simulink model "mrefrobotarm_modified_previous_y_previous_ref"  (R2018b)
settings: Solver=FixedStepAuto  StartTime=0.0  StopTime=60  RelTol=1e-3  AbsTol=1e-6
undefined symbols (not defined in the file or in its folder): sfunxy2
libraries: neural x301, simulink x1
(part 8 of 10)

== system mrefrobotarm_modified_previous_y_previous_ref/Feed-Forward Neural Network5/Layer 2/Delays 1 ==
  "p{2}" : Inport  PortDimensions=64
      mask Display: e = 0.06;c1 = [120 230 180]/255;c2 = ([120 230 180]+0)/(256+128);c3 = ([120 230 180]+128)/(256+128);patch([0 1 1 0],[0 0 1 1],c1);patch([0 1 1 1-e 1-e 0+e],[0 0 1 1-e 0+e 0+e],c2);patch([0 0 1 1-e 0+e 0+e],[0 1 1 1-e 1-e 0+e],c3);plot([0 1 1 0 0],[0 0 1 1 0]);
  mux : Mux  Inputs=1
      mask Display: e = 0.06;c1 = [120 150 230]/255;c2 = ([120 150 230]+0)/383;c3 = ([120 150 230]+128)/383;patch([0 1 1 0],[0 0 1 1],c1);patch([0 1 1 1-e 1-e 0+e],[0 0 1 1-e 0+e 0+e],c2);patch([0 0 1 1-e 0+e 0+e],[0 1 1 1-e 1-e 0+e],c3);plot([0 1 1 0 0],[0 0 1 1 0]);disp('Mux')
  "pd{2,1}" : Outport
      mask Display: e = 0.06;c1 = [120 230 180]/255;c2 = ([120 230 180]+0)/(256+128);c3 = ([120 230 180]+128)/(256+128);patch([0 1 1 0],[0 0 1 1],c1);patch([0 1 1 1-e 1-e 0+e],[0 0 1 1-e 0+e 0+e],c2);patch([0 0 1 1-e 0+e 0+e],[0 1 1 1-e 1-e 0+e],c3);plot([0 1 1 0 0],[0 0 1 1 0]);
  wires:
  "p{2}"/1 -> mux/1
  mux/1 -> "pd{2,1}"/1

== system mrefrobotarm_modified_previous_y_previous_ref/Feed-Forward Neural Network5/Layer 2/LW{2,1} ==
  "ad{2,1}" : Inport  PortDimensions=64
      mask Display: e = 0.06;c1 = [120 230 180]/255;c2 = ([120 230 180]+0)/(256+128);c3 = ([120 230 180]+128)/(256+128);patch([0 1 1 0],[0 0 1 1],c1);patch([0 1 1 1-e 1-e 0+e],[0 0 1 1-e 0+e 0+e],c2);patch([0 0 1 1-e 0+e 0+e],[0 1 1 1-e 1-e 0+e],c3);plot([0 1 1 0 0],[0 0 1 1 0]);
  "IW{2,1}(1,:)'" : Constant  Value=[0.1342055289137980278457717986384523101150989532470703125;-0.286006926010919482195049567962996661663055419921875;-0.189584300225614732493539804636384360492229461669921875;-0.09398592052439856681100849300491972826421260833740234375;-0.0188392157778938286460945761291441158391535282135009765625;-0.1923501339435728929583291346716578118503093719482421875;0.238509813288973526734793040304793976247310638427734375;0.11951515110633703642406544531695544719696044921875;0.204186071860302853497870501087163574993610382080078125;0.5849411103638357811718151424429379403591156005859375;0.1950905033324568937924681222284561954438686370849609375;0.1062361826918395701913055972909205593168735504150390625;-0.200821513449202626588885323144495487213134765625;-0.19738416598699581872011776795261539518833160400390625;0.71704659511815471706341895696823485195636749267578125;-0.00549944375120274032975320466221091919578611850738525390625;-0.235512717208835986593129518951172940433025360107421875;-0.039067003473963766990717516591757885180413722991943359375;0.043539011617688715138907440405091620050370693206787109375;0.0182914099974050940733416581451820093207061290740966796875;-0.334218590430510886779558177295257337391376495361328125;0.26028297183638426925966768976650200784206390380859375;-0.06186171849779309450667597047868184745311737060546875;-0.044099441791101867682556303407181985676288604736328125;-0.044511577979650100711506155448660138063132762908935546875;0.119555008380753780006244824107852764427661895751953125;0.0975331942480585356580746747567900456488132476806640625;0.14401308110082655655759253932046703994274139404296875;0.09857621208828577785698854540896718390285968780517578125;0.47497175248592171659112182169337756931781768798828125;0.384151718188493251915360815473832190036773681640625;0.08918730933547781847270385924275615252554416656494140625;0.07368007693144344727453898258318076841533184051513671875;-0.04662287957187867537545145069088903255760669708251953125;-0.05534159155879812830303166037992923520505428314208984375;-0.034731517165705348693105491975074983201920986175537109375;-0.0658721352210664135018447495895088650286197662353515625;-0.10086130490396698344834902627553674392402172088623046875;0.003373147010439256181235645470906092668883502483367919921875;-0.2031346185319345687414482881649746559560298919677734375;0.1486614292603463394204510450435918755829334259033203125;-0.09620946865737722841771528692333959043025970458984375;-0.0937563823852701483385629899203195236623287200927734375;-0.048708045774094189950265132438289583660662174224853515625;-0.284382094020042275328563619041233323514461517333984375;-0.086738788145810097329757581974263302981853485107421875;0.032848985855427038915710369337830343283712863922119140625;0.013815272864861678769887731732524116523563861846923828125;-0.0234293323723167266903200101069160155020654201507568359375;0.488525039842316710636538346079760231077671051025390625;0.142263860904981165322880087842349894344806671142578125;0.354491458796687697319072185564436949789524078369140625;0.07703656948803112858303876464560744352638721466064453125;-0.226657802141436770515525722657912410795688629150390625;-0.01280840630040126597311012091040538507513701915740966796875;-0.3813405138040832920154343810281716287136077880859375;-0.0872216781847491018364593173828325234353542327880859375;-0.07378247722757168280960371475885040126740932464599609375;0.277010557469474283376342782503343187272548675537109375;-0.2319499909931690695419348458017338998615741729736328125;0.435196146956528362448324287470313720405101776123046875;-0.10238856342738970883754490159844863228499889373779296875;-0.1313325295288241545410556909700972028076648712158203125;-0.05219163910958524166261440768721513450145721435546875]
      mask Display: e = 0.06;c1 = [120 150 230]/255;c2 = ([120 150 230]+0)/383;c3 = ([120 150 230]+128)/383;patch([0 1 1 0],[0 0 1 1],c1);patch([0 1 1 1-e 1-e 0+e],[0 0 1 1-e 0+e 0+e],c2);patch([0 0 1 1-e 0+e 0+e],[0 1 1 1-e 1-e 0+e],c3);plot([0 1 1 0 0],[0 0 1 1 0]);disp('weights');
  Mux : Mux  Inputs=1
      mask Display: e = 0.06;c1 = [120 150 230]/255;c2 = ([120 150 230]+0)/383;c3 = ([120 150 230]+128)/383;patch([0 1 1 0],[0 0 1 1],c1);patch([0 1 1 1-e 1-e 0+e],[0 0 1 1-e 0+e 0+e],c2);patch([0 0 1 1-e 0+e 0+e],[0 1 1 1-e 1-e 0+e],c3);plot([0 1 1 0 0],[0 0 1 1 0]);disp('Mux');
  dotprod1 : neural/Weight Functions/dotprod
  "lz{2,1}" : Outport
      mask Display: e = 0.06;c1 = [120 230 180]/255;c2 = ([120 230 180]+0)/(256+128);c3 = ([120 230 180]+128)/(256+128);patch([0 1 1 0],[0 0 1 1],c1);patch([0 1 1 1-e 1-e 0+e],[0 0 1 1-e 0+e 0+e],c2);patch([0 0 1 1-e 0+e 0+e],[0 1 1 1-e 1-e 0+e],c3);plot([0 1 1 0 0],[0 0 1 1 0]);
  wires:
  "IW{2,1}(1,:)'"/1 -> dotprod1/1
  "ad{2,1}"/1 -> dotprod1/2
  dotprod1/1 -> Mux/1
  Mux/1 -> "lz{2,1}"/1

== system mrefrobotarm_modified_previous_y_previous_ref/small_error/Layer 1/Delays 1 ==
  "p{1}" : Inport  PortDimensions=8
      mask Display: e = 0.06;c1 = [120 230 180]/255;c2 = ([120 230 180]+0)/(256+128);c3 = ([120 230 180]+128)/(256+128);patch([0 1 1 0],[0 0 1 1],c1);patch([0 1 1 1-e 1-e 0+e],[0 0 1 1-e 0+e 0+e],c2);patch([0 0 1 1-e 0+e 0+e],[0 1 1 1-e 1-e 0+e],c3);plot([0 1 1 0 0],[0 0 1 1 0]);
  mux : Mux  Inputs=1
      mask Display: e = 0.06;c1 = [120 150 230]/255;c2 = ([120 150 230]+0)/383;c3 = ([120 150 230]+128)/383;patch([0 1 1 0],[0 0 1 1],c1);patch([0 1 1 1-e 1-e 0+e],[0 0 1 1-e 0+e 0+e],c2);patch([0 0 1 1-e 0+e 0+e],[0 1 1 1-e 1-e 0+e],c3);plot([0 1 1 0 0],[0 0 1 1 0]);disp('Mux')
  "pd{1,1}" : Outport
      mask Display: e = 0.06;c1 = [120 230 180]/255;c2 = ([120 230 180]+0)/(256+128);c3 = ([120 230 180]+128)/(256+128);patch([0 1 1 0],[0 0 1 1],c1);patch([0 1 1 1-e 1-e 0+e],[0 0 1 1-e 0+e 0+e],c2);patch([0 0 1 1-e 0+e 0+e],[0 1 1 1-e 1-e 0+e],c3);plot([0 1 1 0 0],[0 0 1 1 0]);
  wires:
  "p{1}"/1 -> mux/1
  mux/1 -> "pd{1,1}"/1
